simulink model "model"  (R2020b)
settings: Solver=VariableStepAuto  StartTime=0.0  StopTime=10.0  RelTol=1e-3
settings Model: Creator=SAGAR  LastModifiedBy=SAGAR

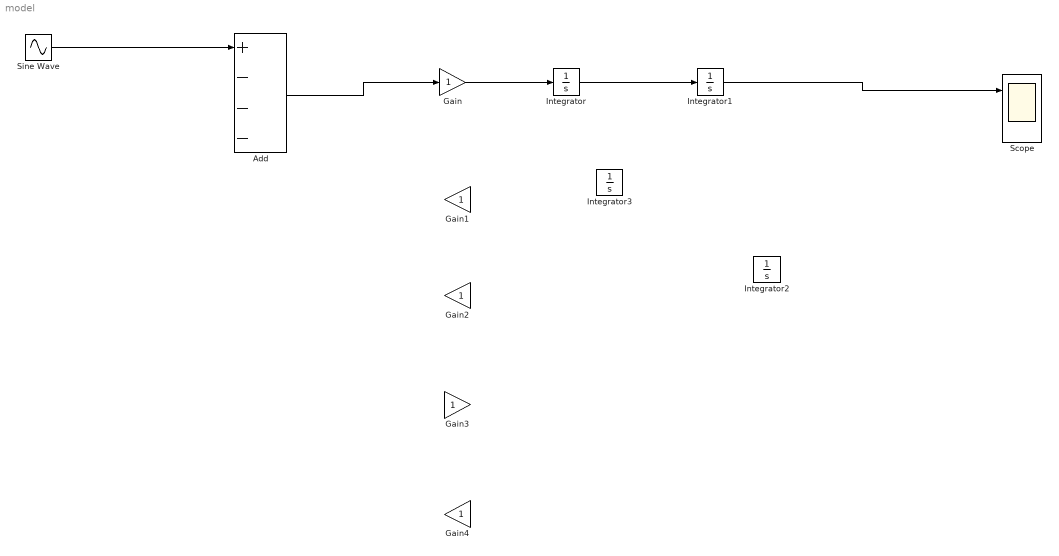
== system model ==
  Add : Sum  Inputs=+---
  Gain{,1..4} (5 alike) : Gain
  Integrator{,1..3} (4 alike) : Integrator
  Scope : Scope  NumInputPorts=2
  Sine Wave : Sin  SampleTime=0
  wires:
  Sine Wave/1 -> Add/1
  Integrator/1 -> Integrator1/1
  Gain/1 -> Integrator/1
  Add/1 -> Gain/1
  Integrator1/1 -> Scope/1
